simulink model "robusnost_nelin_sim"  (R2020a)
settings: Solver=ode5  StartTime=0.0  StopTime=tfin  FixedStep=1e-4  RelTol=1e-3
values from neighbouring files (symbols this model uses):
  F = Fe    [robusnost_nelin_sim_matlab.m]
  F_initial = mi_initial*V    [robusnost_nelin_sim_matlab.m]
  K1 = 0.03    [robusnost_nelin_sim_matlab.m]
  K2 = 0.5    [robusnost_nelin_sim_matlab.m]
  mi_max = 1    [robusnost_nelin_sim_matlab.m]
  SF = 10    [robusnost_nelin_sim_matlab.m]
  V = 4    [robusnost_nelin_sim_matlab.m]
  x10 = X_initial    [robusnost_nelin_sim_matlab.m]
  x20 = S_initial    [robusnost_nelin_sim_matlab.m]
  Y = 0.5    [robusnost_nelin_sim_matlab.m]
  Y1 = Y - 0.2*Y    (= 0.4)    [robusnost_nelin_sim_matlab.m]
  Y2 = Y - 0.1*Y    (= 0.45)    [robusnost_nelin_sim_matlab.m]
  Y3 = Y + 0.1*Y    (= 0.55)    [robusnost_nelin_sim_matlab.m]
  Y4 = Y + 0.2*Y    (= 0.6)    [robusnost_nelin_sim_matlab.m]
undefined symbols (not defined in the file or in its folder): magnitude
settings Model: Creator=anaMceranic  LastModifiedBy=anaMceranic
settings DataIOCC: ReturnWorkspaceOutputs=off

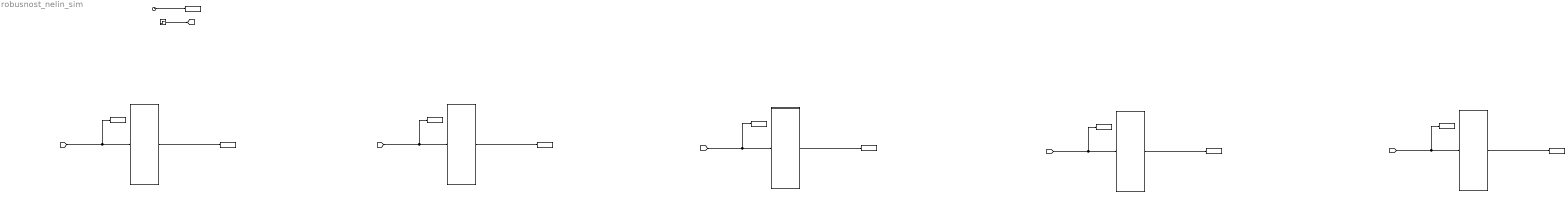
== system robusnost_nelin_sim ==
  note: nominalni Y
  note: 0.8 Y
  note: 0.9 Y
  note: 1.1 Y
  note: 1.2 Y
  note: Nelinearni sistem, otvorena sprega, ispitivanje robusnosti
      | Prelazak iz početnog stanja u ravnotežno
  Clock : Clock
  F : Step  Time=0  Before=F_initial  After=F  SampleTime=0
  Subsystem1 : Subsystem
  Subsystem2 : Subsystem
  Subsystem3 : Subsystem
  Subsystem4 : Subsystem
  Subsystem5 : Subsystem
  To Workspace1 : ToWorkspace  VariableName=t_out  SampleTime=-1
  To Workspace10 : ToWorkspace  VariableName=S_out4  SampleTime=-1
  To Workspace11 : ToWorkspace  VariableName=F_out4  SampleTime=-1
  To Workspace2 : ToWorkspace  VariableName=S_out1  SampleTime=-1
  To Workspace3 : ToWorkspace  VariableName=S_out  SampleTime=-1
  To Workspace4 : ToWorkspace  VariableName=F_out  SampleTime=-1
  To Workspace5 : ToWorkspace  VariableName=F_out1  SampleTime=-1
  To Workspace6 : ToWorkspace  VariableName=S_out2  SampleTime=-1
  To Workspace7 : ToWorkspace  VariableName=F_out2  SampleTime=-1
  To Workspace8 : ToWorkspace  VariableName=S_out3  SampleTime=-1
  To Workspace9 : ToWorkspace  VariableName=F_out3  SampleTime=-1
  wires:
  Clock/1 -> To Workspace1/1
  F/1 -> [F]
  [F] -> To Workspace4/1, Subsystem1/1(u)
  Subsystem1/1(y) -> To Workspace3/1
  [F] -> To Workspace5/1, Subsystem2/1(u)
  Subsystem2/1(y) -> To Workspace2/1
  [F] -> To Workspace7/1, Subsystem3/1(u)
  Subsystem3/1(y) -> To Workspace6/1
  [F] -> To Workspace9/1, Subsystem4/1(u)
  Subsystem4/1(y) -> To Workspace8/1
  [F] -> To Workspace11/1, Subsystem5/1(u)
  Subsystem5/1(y) -> To Workspace10/1

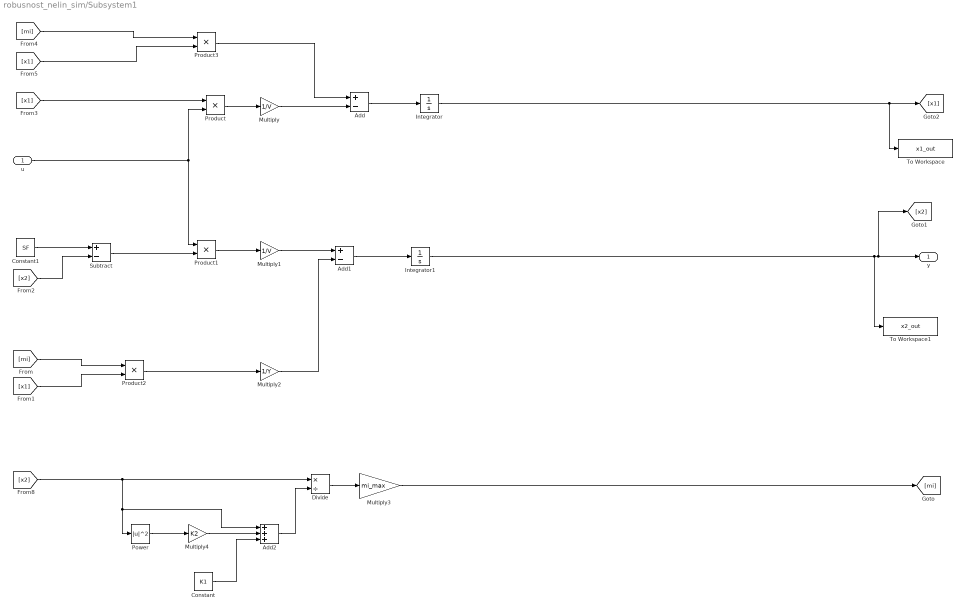
== system robusnost_nelin_sim/Subsystem1 ==
  u : Inport
  Add : Sum  Inputs=+-
  Add1 : Sum  Inputs=+-
  Add2 : Sum  Inputs=+++
  Constant : Constant  Value=K1
  Constant1 : Constant  Value=SF
  Divide : Product  Inputs=*/
  Integrator : Integrator  InitialCondition=x10
  Integrator1 : Integrator  InitialCondition=x20
  Multiply : Gain  Gain=1/V
  Multiply1 : Gain  Gain=1/V
  Multiply2 : Gain  Gain=1/Y
  Multiply3 : Gain  Gain=mi_max
  Multiply4 : Gain  Gain=K2
  Power : Math  Operator=magnitude^2  SaturateOnIntegerOverflow=on
  Product{,1..3} (4 alike) : Product
  Subtract : Sum  Inputs=+-
  To Workspace : ToWorkspace  VariableName=x1_out  SampleTime=-1
  To Workspace1 : ToWorkspace  VariableName=x2_out  SampleTime=-1
  y : Outport
  wires:
  [x1] -> Product2/2
  Product2/1 -> Multiply2/1
  Multiply/1 -> Add/2
  Add2/1 -> Divide/2
  Constant/1 -> Add2/3
  [x1] -> Product3/2
  Multiply4/1 -> Add2/2
  [mi] -> Product2/1
  Multiply3/1 -> [mi]
  Power/1 -> Multiply4/1
  Constant1/1 -> Subtract/1
  [x2] -> Subtract/2
  Add1/1 -> Integrator1/1
  Multiply2/1 -> Add1/2
  Integrator1/1 -> [x2], y/1, To Workspace1/1
  Divide/1 -> Multiply3/1
  Integrator/1 -> [x1], To Workspace/1
  Product3/1 -> Add/1
  u/1 -> Product1/1, Product/2
  [x1] -> Product/1
  Multiply1/1 -> Add1/1
  Product1/1 -> Multiply1/1
  Subtract/1 -> Product1/2
  [x2] -> Divide/1, Add2/1, Power/1
  Add/1 -> Integrator/1
  Product/1 -> Multiply/1
  [mi] -> Product3/1

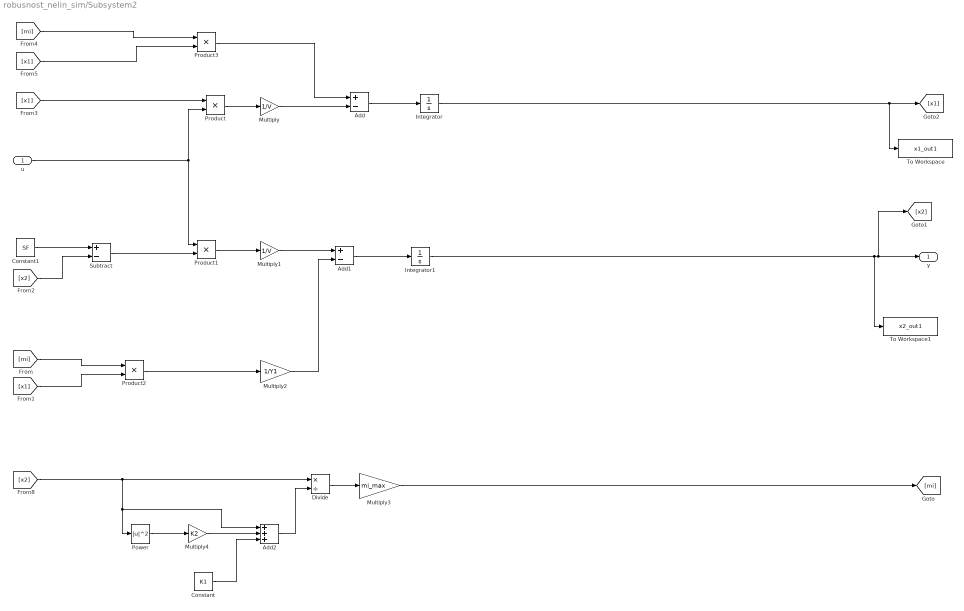
== system robusnost_nelin_sim/Subsystem2 ==
  u : Inport
  Add : Sum  Inputs=+-
  Add1 : Sum  Inputs=+-
  Add2 : Sum  Inputs=+++
  Constant : Constant  Value=K1
  Constant1 : Constant  Value=SF
  Divide : Product  Inputs=*/
  Integrator : Integrator  InitialCondition=x10
  Integrator1 : Integrator  InitialCondition=x20
  Multiply : Gain  Gain=1/V
  Multiply1 : Gain  Gain=1/V
  Multiply2 : Gain  Gain=1/Y1
  Multiply3 : Gain  Gain=mi_max
  Multiply4 : Gain  Gain=K2
  Power : Math  Operator=magnitude^2  SaturateOnIntegerOverflow=on
  Product{,1..3} (4 alike) : Product
  Subtract : Sum  Inputs=+-
  To Workspace : ToWorkspace  VariableName=x1_out1  SampleTime=-1
  To Workspace1 : ToWorkspace  VariableName=x2_out1  SampleTime=-1
  y : Outport
  wires:
  [x1] -> Product2/2
  Product2/1 -> Multiply2/1
  Multiply/1 -> Add/2
  Add2/1 -> Divide/2
  Constant/1 -> Add2/3
  [x1] -> Product3/2
  Multiply4/1 -> Add2/2
  [mi] -> Product2/1
  Multiply3/1 -> [mi]
  Power/1 -> Multiply4/1
  Constant1/1 -> Subtract/1
  [x2] -> Subtract/2
  Add1/1 -> Integrator1/1
  Multiply2/1 -> Add1/2
  Integrator1/1 -> [x2], y/1, To Workspace1/1
  Divide/1 -> Multiply3/1
  Integrator/1 -> [x1], To Workspace/1
  Product3/1 -> Add/1
  u/1 -> Product1/1, Product/2
  [x1] -> Product/1
  Multiply1/1 -> Add1/1
  Product1/1 -> Multiply1/1
  Subtract/1 -> Product1/2
  [x2] -> Divide/1, Add2/1, Power/1
  Add/1 -> Integrator/1
  Product/1 -> Multiply/1
  [mi] -> Product3/1

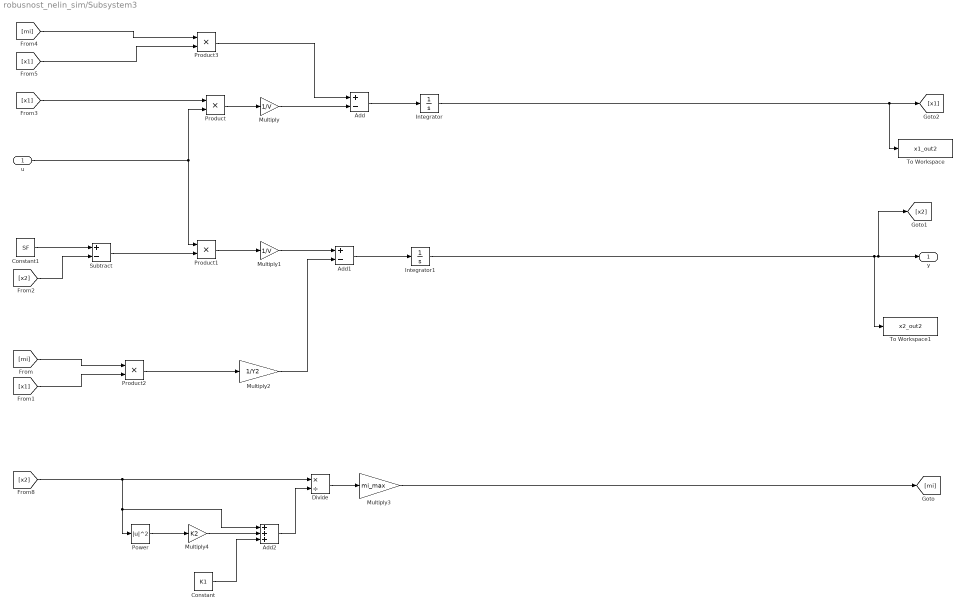
== system robusnost_nelin_sim/Subsystem3 ==
  u : Inport
  Add : Sum  Inputs=+-
  Add1 : Sum  Inputs=+-
  Add2 : Sum  Inputs=+++
  Constant : Constant  Value=K1
  Constant1 : Constant  Value=SF
  Divide : Product  Inputs=*/
  Integrator : Integrator  InitialCondition=x10
  Integrator1 : Integrator  InitialCondition=x20
  Multiply : Gain  Gain=1/V
  Multiply1 : Gain  Gain=1/V
  Multiply2 : Gain  Gain=1/Y2
  Multiply3 : Gain  Gain=mi_max
  Multiply4 : Gain  Gain=K2
  Power : Math  Operator=magnitude^2  SaturateOnIntegerOverflow=on
  Product{,1..3} (4 alike) : Product
  Subtract : Sum  Inputs=+-
  To Workspace : ToWorkspace  VariableName=x1_out2  SampleTime=-1
  To Workspace1 : ToWorkspace  VariableName=x2_out2  SampleTime=-1
  y : Outport
  wires:
  [x1] -> Product2/2
  Product2/1 -> Multiply2/1
  Multiply/1 -> Add/2
  Add2/1 -> Divide/2
  Constant/1 -> Add2/3
  [x1] -> Product3/2
  Multiply4/1 -> Add2/2
  [mi] -> Product2/1
  Multiply3/1 -> [mi]
  Power/1 -> Multiply4/1
  Constant1/1 -> Subtract/1
  [x2] -> Subtract/2
  Add1/1 -> Integrator1/1
  Multiply2/1 -> Add1/2
  Integrator1/1 -> [x2], y/1, To Workspace1/1
  Divide/1 -> Multiply3/1
  Integrator/1 -> [x1], To Workspace/1
  Product3/1 -> Add/1
  u/1 -> Product1/1, Product/2
  [x1] -> Product/1
  Multiply1/1 -> Add1/1
  Product1/1 -> Multiply1/1
  Subtract/1 -> Product1/2
  [x2] -> Divide/1, Add2/1, Power/1
  Add/1 -> Integrator/1
  Product/1 -> Multiply/1
  [mi] -> Product3/1

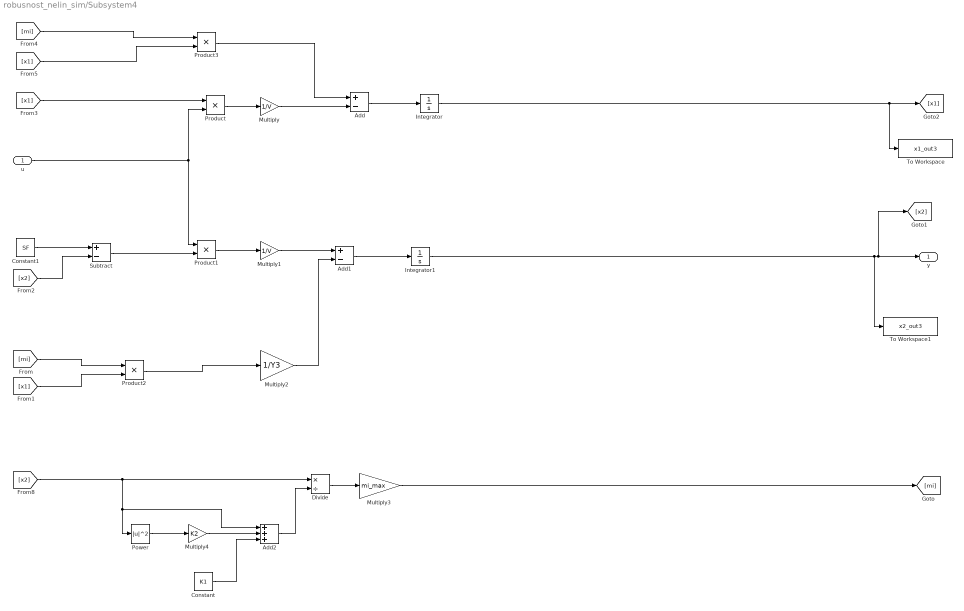
== system robusnost_nelin_sim/Subsystem4 ==
  u : Inport
  Add : Sum  Inputs=+-
  Add1 : Sum  Inputs=+-
  Add2 : Sum  Inputs=+++
  Constant : Constant  Value=K1
  Constant1 : Constant  Value=SF
  Divide : Product  Inputs=*/
  Integrator : Integrator  InitialCondition=x10
  Integrator1 : Integrator  InitialCondition=x20
  Multiply : Gain  Gain=1/V
  Multiply1 : Gain  Gain=1/V
  Multiply2 : Gain  Gain=1/Y3
  Multiply3 : Gain  Gain=mi_max
  Multiply4 : Gain  Gain=K2
  Power : Math  Operator=magnitude^2  SaturateOnIntegerOverflow=on
  Product{,1..3} (4 alike) : Product
  Subtract : Sum  Inputs=+-
  To Workspace : ToWorkspace  VariableName=x1_out3  SampleTime=-1
  To Workspace1 : ToWorkspace  VariableName=x2_out3  SampleTime=-1
  y : Outport
  wires:
  [x1] -> Product2/2
  Product2/1 -> Multiply2/1
  Multiply/1 -> Add/2
  Add2/1 -> Divide/2
  Constant/1 -> Add2/3
  [x1] -> Product3/2
  Multiply4/1 -> Add2/2
  [mi] -> Product2/1
  Multiply3/1 -> [mi]
  Power/1 -> Multiply4/1
  Constant1/1 -> Subtract/1
  [x2] -> Subtract/2
  Add1/1 -> Integrator1/1
  Multiply2/1 -> Add1/2
  Integrator1/1 -> [x2], y/1, To Workspace1/1
  Divide/1 -> Multiply3/1
  Integrator/1 -> [x1], To Workspace/1
  Product3/1 -> Add/1
  u/1 -> Product1/1, Product/2
  [x1] -> Product/1
  Multiply1/1 -> Add1/1
  Product1/1 -> Multiply1/1
  Subtract/1 -> Product1/2
  [x2] -> Divide/1, Add2/1, Power/1
  Add/1 -> Integrator/1
  Product/1 -> Multiply/1
  [mi] -> Product3/1

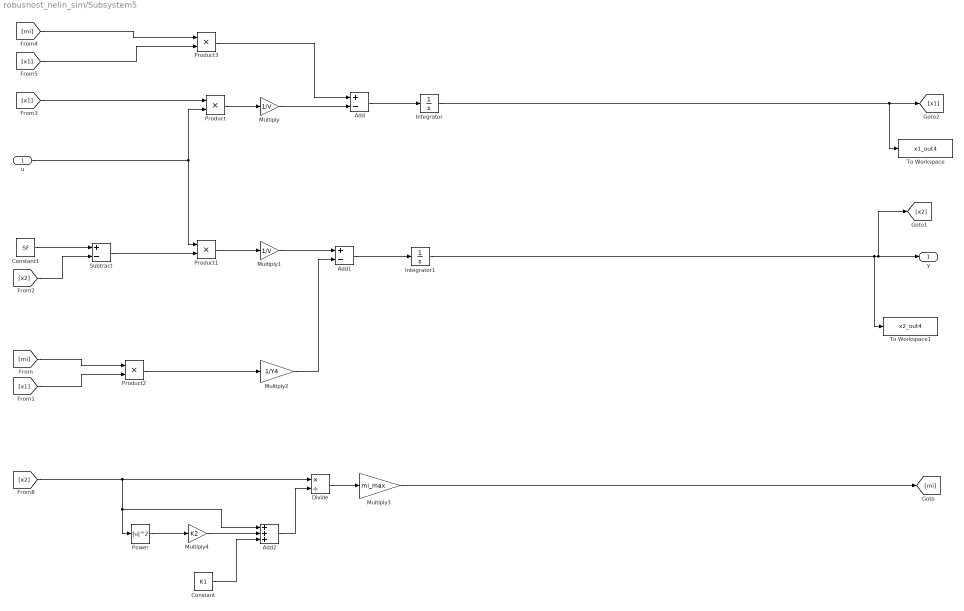
== system robusnost_nelin_sim/Subsystem5 ==
  u : Inport
  Add : Sum  Inputs=+-
  Add1 : Sum  Inputs=+-
  Add2 : Sum  Inputs=+++
  Constant : Constant  Value=K1
  Constant1 : Constant  Value=SF
  Divide : Product  Inputs=*/
  Integrator : Integrator  InitialCondition=x10
  Integrator1 : Integrator  InitialCondition=x20
  Multiply : Gain  Gain=1/V
  Multiply1 : Gain  Gain=1/V
  Multiply2 : Gain  Gain=1/Y4
  Multiply3 : Gain  Gain=mi_max
  Multiply4 : Gain  Gain=K2
  Power : Math  Operator=magnitude^2  SaturateOnIntegerOverflow=on
  Product{,1..3} (4 alike) : Product
  Subtract : Sum  Inputs=+-
  To Workspace : ToWorkspace  VariableName=x1_out4  SampleTime=-1
  To Workspace1 : ToWorkspace  VariableName=x2_out4  SampleTime=-1
  y : Outport
  wires:
  [x1] -> Product2/2
  Product2/1 -> Multiply2/1
  Multiply/1 -> Add/2
  Add2/1 -> Divide/2
  Constant/1 -> Add2/3
  [x1] -> Product3/2
  Multiply4/1 -> Add2/2
  [mi] -> Product2/1
  Multiply3/1 -> [mi]
  Power/1 -> Multiply4/1
  Constant1/1 -> Subtract/1
  [x2] -> Subtract/2
  Add1/1 -> Integrator1/1
  Multiply2/1 -> Add1/2
  Integrator1/1 -> [x2], y/1, To Workspace1/1
  Divide/1 -> Multiply3/1
  Integrator/1 -> [x1], To Workspace/1
  Product3/1 -> Add/1
  u/1 -> Product1/1, Product/2
  [x1] -> Product/1
  Multiply1/1 -> Add1/1
  Product1/1 -> Multiply1/1
  Subtract/1 -> Product1/2
  [x2] -> Divide/1, Add2/1, Power/1
  Add/1 -> Integrator/1
  Product/1 -> Multiply/1
  [mi] -> Product3/1
